simulink model "imctmpl"  (Simulink 10.1)
settings: Solver=ode45  StartTime=0.0  StopTime=1600  RelTol=1e-3  EnableMultiTasking=on
PreLoadFcn:
  | variables
values from neighbouring files (symbols this model uses):
  Kp = 1.05    [variables.m]
  T1p = 139.41    [variables.m]
  T2p = 14.29    [variables.m]
  thetap = 9.07    [variables.m]
  Ts = 1    [variables.m]
undefined symbols (not defined in the file): demi_serie, serie, set_up
libraries: simulink x1
settings Model: Creator=auto2  LastModifiedBy=aif  ExtModeTrigMode=oneshot  ExtModeArmWhenConnect=off
settings DataIOCC: SignalLoggingSaveFormat=ModelDataLogs  SaveOutput=off  SaveTime=off  SignalLoggingName=sigsOut
settings OptimizationCC: BooleanDataType=off  ExpressionDepthLimit=2147483647  InitFltsAndDblsToZero=on
settings DebuggingCC: SaveWithParameterizedLinksMsg=none  SignalResolutionControl=TryResolveAllWithWarning  MultiTaskDSMMsg=warning  MultiTaskCondExecSysMsg=none  FcnCallInpInsideContextMsg=warning  StateNameClashWarn=warning
settings HardwareCC: TargetUnknown=on
settings ConfigComp: CovSFcnEnable=off

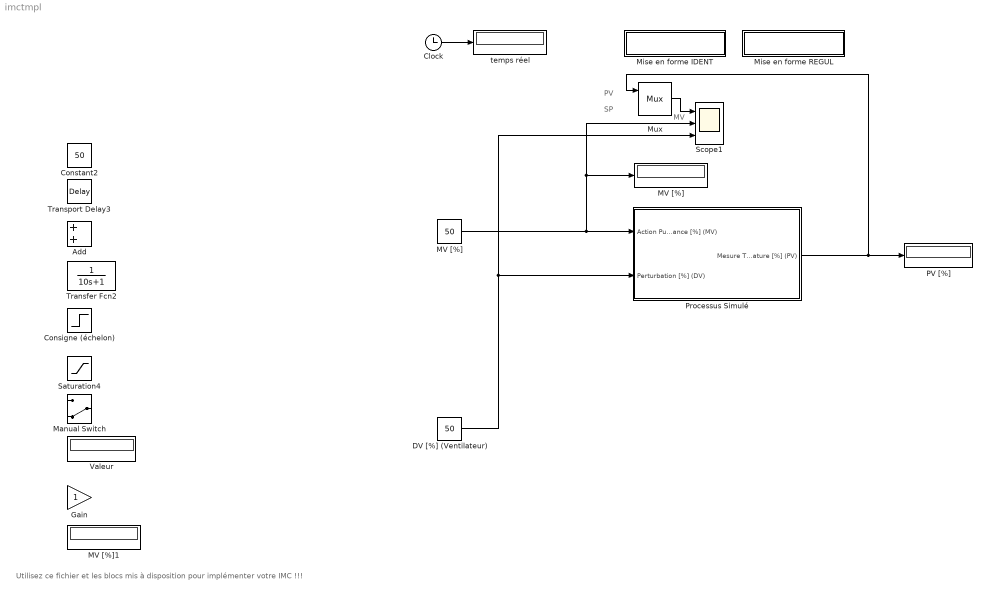
== system imctmpl ==
  note: PV
  note: SP
  note: MV
  note: Utilisez ce fichier et les blocs mis à disposition pour implémenter votre IMC !!!
  Add : Sum  StartFcn=simu(1,1).bloc_Add='labo'
  Clock : Clock
      settings: StartFcn=simu(1,1).bloc_Clock='labo'
  Consigne (échelon) : Step  StartFcn=simu(1,1).bloc_Step='labo'  Time=100  Before=50  After=50  SampleTime=0
  Constant2 : Constant  StartFcn=simu(1,1).bloc_cst='labo'  Value=50
  DV [%] (Ventilateur) : Constant  StartFcn=simu(1,1).bloc_DV='labo'  Value=50
  Gain : Gain  StartFcn=simu(1,1).bloc_Gain='labo'
  MV [%] : Constant  StartFcn=simu(1,1).bloc_MV='labo'  Value=50
  "MV [%] " : Display
      settings: StartFcn=simu(1,1).bloc_Display_MV='labo'
  MV [%]1 : Display
      settings: StartFcn=simu(1,1).bloc_Display_MV='labo'
  Manual Switch : ManualSwitch  StartFcn=simu(1,1).bloc_Switch='labo'  CurrentSetting=0
  Mise en forme IDENT : Subsystem
      settings: OpenFcn=|
      | t=Scope_imc.time;A=[Scope_imc.signals.values];
      | y=A(:,1);u=A(:,3);
      | subplot(211)
      | plot(t,u,'black');
      | title('MV')
      | subplot(212)
      | plot(t,y,'black');
      | title('PV')
      | grid;figure(gcf)
      mask Display: disp('Mise en forme IDENT')
  Mise en forme REGUL : Subsystem
      settings: OpenFcn=|
      | t=Scope_imc.time;
      | A=[Scope_imc.signals.values];
      | y=A(:,1);
      | ysp=A(:,2);
      | u=A(:,3);
      | figure;
      | subplot(211);
      | plot(t,y,'black',t,ysp,'black');
      | grid;
      | title('PV [%] et SP [%]');
      | subplot(212),
      | plot(t,u,'black');
      | grid;
      | figure(gcf);
      | title('MV [%]')
      mask Display: disp('Mise en forme REGUL');
  Mux : Mux  StartFcn=simu(1,1).bloc_Mux='labo'  Inputs=2
  PV [%] : Display
      settings: StartFcn=simu(1,1).bloc_Display_PV='labo'
  Processus Simulé : Subsystem  StartFcn=simu(1).bloc_Process='labo'  mask{set_up=set_up, serie=serie, demi_serie=demi_serie}
      mask prompts: serie "Série"; demi_serie "Demi série"
      mask init:
      | %%%%%%%%%%%%%%%%%%%%%%%%%%%%%%%%%
      | 
      | switch set_up
      |    case 1
      |         Kd = -0.64;
      |         T1d = 81.54;
      |         T2d = 18.9;
      |         thetad = 12.49;
      |    case 2
      |         Kd = -0.43;
      |         T1d = 34.66;
      |         T2d = 1.13;
      |         thetad = 6.08; 
      |     case 3
      |         Kd = -0.34;
      |         T1d = 82.52;
      |         T2d = 20.99;
      |         thetad = 8.42;  
      | end
      | 
      | if (demi_serie == 'A')
      |     dserie = 1;
      | else
      |     dserie = 5;
      | end    
      | 
      | seed = str2num([num2str(serie) num2str(serie) num2str(dserie) num2str(set_up)]);
      | 
      | rng(seed)
      | x1 = (rand - 1)/5;
      | rng(seed+1)
      | x2 = (rand - 1)/5;
      | rng(seed+2)
      | x3 = (rand - 1)/5;
      | rng(seed+3)
      | x4 = (rand - 1)/5;
      | 
      | Kd = Kd*(1+x1);
      | T1d = T1d*(1+x2);
      | T2d = T2d*(1+x3);
      | thetad =thetad*(1+x4);
  Saturation4 : Saturate  StartFcn=simu(1,1).bloc_Sat='labo'  UpperLimit=100  LowerLimit=0
  Scope1 : Scope  NumInputPorts=3
      settings: StartFcn=simu(1,1).bloc_Scope='labo'
  Transfer Fcn2 : TransferFcn  StartFcn=simu(1,1).bloc_TF='labo'  Denominator=[10 1]
  Transport Delay3 : TransportDelay  StartFcn=simu(1,1).bloc_Delay='labo'  DelayTime=0.1
  Valeur : Display
      settings: StartFcn=simu(1,1).bloc_Display='labo'
  temps réel : Display
      settings: StartFcn=simu(1,1).bloc_Display_Clock='labo'
  wires:
  Mux/1 -> Scope1/1
  MV [%]/1 -> Processus Simulé/1(Action Puissance [%] (MV)), Scope1/2, "MV [%] "/1
  Processus Simulé/1(Mesure Température [%] (PV)) -> Mux/1, PV [%]/1
  DV [%] (Ventilateur)/1 -> Processus Simulé/2(Perturbation [%] (DV)), Scope1/3
  Clock/1 -> temps réel/1

== system imctmpl/Mise en forme IDENT ==

== system imctmpl/Mise en forme REGUL ==

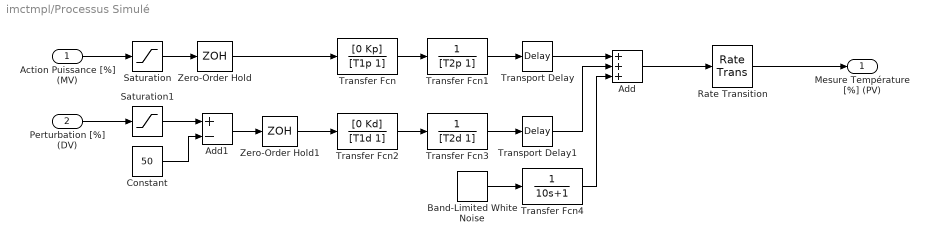
== system imctmpl/Processus Simulé ==
  Action Puissance [%] (MV) : Inport
  Perturbation [%] (DV) : Inport  Port=2
  Add : Sum  Inputs=+++
  Add1 : Sum  Inputs=+-
  Band-Limited White Noise : simulink/Sources/Band-Limited White Noise  Cov=[0.1]  Ts=Ts  seed=[23341]
  Constant : Constant  Value=50  SampleTime=Inf
  Rate Transition : RateTransition  OutPortSampleTime=Ts
  Saturation : Saturate  UpperLimit=100  LowerLimit=0
  Saturation1 : Saturate  UpperLimit=100  LowerLimit=0
  Transfer Fcn : TransferFcn  Numerator=[0 Kp]  Denominator=[T1p 1]
  Transfer Fcn1 : TransferFcn  Numerator=[0 1]  Denominator=[T2p 1]
  Transfer Fcn2 : TransferFcn  Numerator=[0 Kd]  Denominator=[T1d 1]
  Transfer Fcn3 : TransferFcn  Numerator=[0 1]  Denominator=[T2d 1]
  Transfer Fcn4 : TransferFcn  Numerator=[0 1]  Denominator=[10 1]
  Transport Delay : TransportDelay  DelayTime=thetap
  Transport Delay1 : TransportDelay  DelayTime=thetad
  Zero-Order Hold : ZeroOrderHold  SampleTime=Ts
  Zero-Order Hold1 : ZeroOrderHold  SampleTime=Ts
  Mesure Température [%] (PV) : Outport
  wires:
  Transfer Fcn/1 -> Transfer Fcn1/1
  Transfer Fcn1/1 -> Transport Delay/1
  Transport Delay/1 -> Add/1
  Constant/1 -> Add1/2
  Transfer Fcn2/1 -> Transfer Fcn3/1
  Transfer Fcn3/1 -> Transport Delay1/1
  Add1/1 -> Zero-Order Hold1/1
  Add/1 -> Rate Transition/1
  Zero-Order Hold/1 -> Transfer Fcn/1
  Saturation1/1 -> Add1/1
  Saturation/1 -> Zero-Order Hold/1
  Transport Delay1/1 -> Add/2
  Zero-Order Hold1/1 -> Transfer Fcn2/1
  Action Puissance [%] (MV)/1 -> Saturation/1
  Perturbation [%] (DV)/1 -> Saturation1/1
  Rate Transition/1 -> Mesure Température [%] (PV)/1
  Band-Limited White Noise/1 -> Transfer Fcn4/1
  Transfer Fcn4/1 -> Add/3
